simulink model "msim"  (R2024b)
settings: Solver=VariableStepAuto  StartTime=0.0  StopTime=10.0  RelTol=1e-3
values from neighbouring files (symbols this model uses):
  RegStruct = DBReg(dtf)    [db.m]
undefined symbols (not defined in the file or in its folder): dtf
settings Model: Creator=markminerov  LastModifiedBy=markminerov

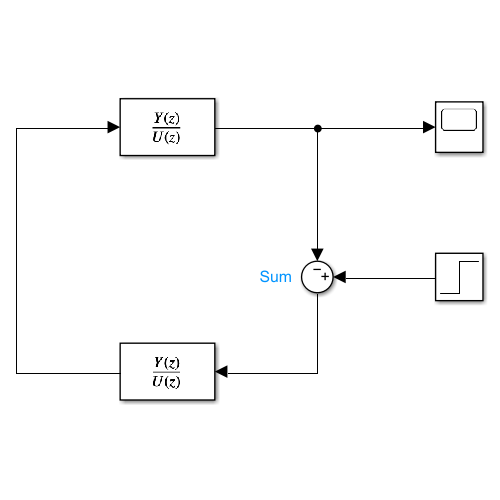
[thumbnail: Simulink's stored preview of the top-level diagram]
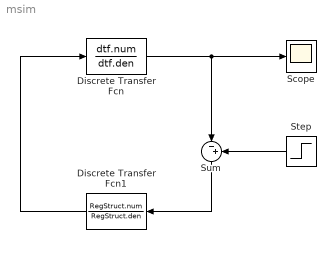
== system msim ==
  Discrete Transfer Fcn : DiscreteTransferFcn  Numerator=dtf.num  Denominator=dtf.den
  Discrete Transfer Fcn1 : DiscreteTransferFcn  Numerator=RegStruct.num  Denominator=RegStruct.den
  Scope : Scope
  Step : Step  SampleTime=0
  Sum : Sum  Inputs=|-+
  wires:
  Discrete Transfer Fcn1/1 -> Discrete Transfer Fcn/1
  Discrete Transfer Fcn/1 -> Sum/1, Scope/1
  Step/1 -> Sum/2
  Sum/1 -> Discrete Transfer Fcn1/1
